simulink model "gm_fft_st"  (R2015a)
settings: Solver=ode45  StartTime=0.0  StopTime=1000.0  RelTol=1e-3
libraries: simulink x3, dspxfrm3 x1, hdlsllib x1
settings Model: CovSFcnEnable=off  Creator=tjia  LastModifiedBy=tjia
settings ConfigSet: ConfigType=Model
settings SolverCC: Priority=auto
settings OptimizationCC: BlockReduction=off  ConditionallyExecuteInputs=off  InlineParamsCompatibleMode=off  UseDivisionForNetSlopeComputation=Off  ForceBlockIOInitOptimize=off  EvaledLifeSpan=Inf  SimCompilerOptimization=Off
settings DebuggingCC: SolverPrmCheckMsg=warning  InheritedTsInSrcMsg=none  AllowSymbolicDim=off  SFMismatchInSimAndRtwBecauseOfMissingDataTypeDiag=warning
settings RTWCC: EnableTagging=off  RTWCompilerOptimization=Off
settings CodeAppCC: ParameterTuningSideEffectCode=Output function  AllmanStyle=off
settings GRTTargetCC: EnableShiftOperators=off  PortableWordSizesTransition=off  GenerateErtSFunctionTransition=off  CreateSILPILBlockTransition=None  CodeProfilingSaveOptionsTransition=SummaryOnly  CodeExecutionProfilingTransition=off  CodeProfilingInstrumentationTransition=off  CodeExecutionProfileVariableTransition=executionProfile  GenerateClassInterface=off

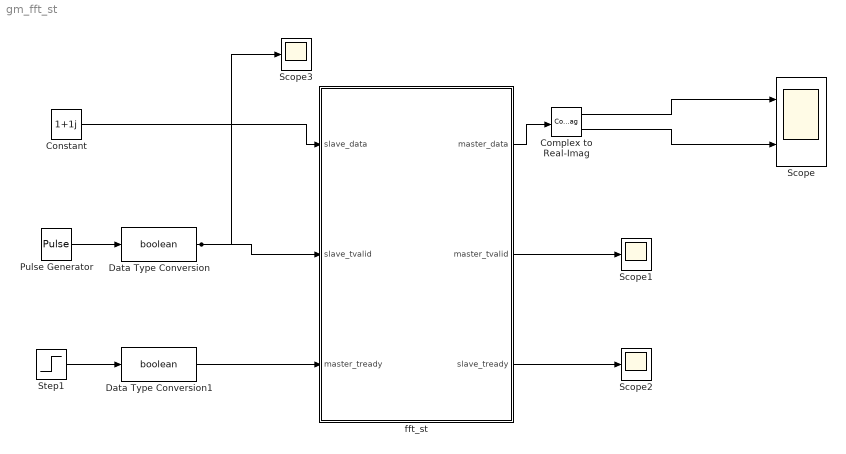
== system gm_fft_st ==
  Complex to Real-Imag : ComplexToRealImag  IOType=none  Commented=off  StatePerturbationForJacobian=1.0e-05
  Constant : Constant  IOType=none  Commented=off  StatePerturbationForJacobian=1.0e-05  Value=1+1j  OutDataTypeStr=int16  SampleTime=1
  Data Type Conversion : DataTypeConversion  IOType=none  Commented=off  StatePerturbationForJacobian=1.0e-05  OutDataTypeStr=boolean
  Data Type Conversion1 : DataTypeConversion  IOType=none  Commented=off  StatePerturbationForJacobian=1.0e-05  OutDataTypeStr=boolean
  Pulse Generator : DiscretePulseGenerator  IOType=none  Commented=off  StatePerturbationForJacobian=1.0e-05  Period=300  PulseWidth=64  PhaseDelay=236
  Scope : Scope  Commented=off  NumInputPorts=2
      settings: IOType=none  StatePerturbationForJacobian=1.0e-05  YMin=-5~-5  YMax=5~5
  Scope1 : Scope  Commented=off
      settings: IOType=none  StatePerturbationForJacobian=1.0e-05
  Scope2 : Scope  Commented=off
      settings: IOType=none  StatePerturbationForJacobian=1.0e-05  SaveName=ScopeData2
  Scope3 : Scope  Commented=off
      settings: IOType=none  StatePerturbationForJacobian=1.0e-05  SaveName=ScopeData3
  Step1 : Step  IOType=none  Commented=off  StatePerturbationForJacobian=1.0e-05  Time=200  SampleTime=1
  fft_st : Subsystem  IOType=none  Commented=off  StatePerturbationForJacobian=1.0e-05  TreatAsAtomicUnit=on
  wires:
  Step1/1 -> Data Type Conversion1/1
  fft_st/3(slave_tready) -> Scope2/1
  Data Type Conversion1/1 -> fft_st/3(master_tready)
  Complex to Real-Imag/2 -> Scope/2
  Complex to Real-Imag/1 -> Scope/1
  fft_st/1(master_data) -> Complex to Real-Imag/1
  Data Type Conversion/1 -> fft_st/2(slave_tvalid), Scope3/1
  fft_st/2(master_tvalid) -> Scope1/1
  Pulse Generator/1 -> Data Type Conversion/1
  Constant/1 -> fft_st/1(slave_data)

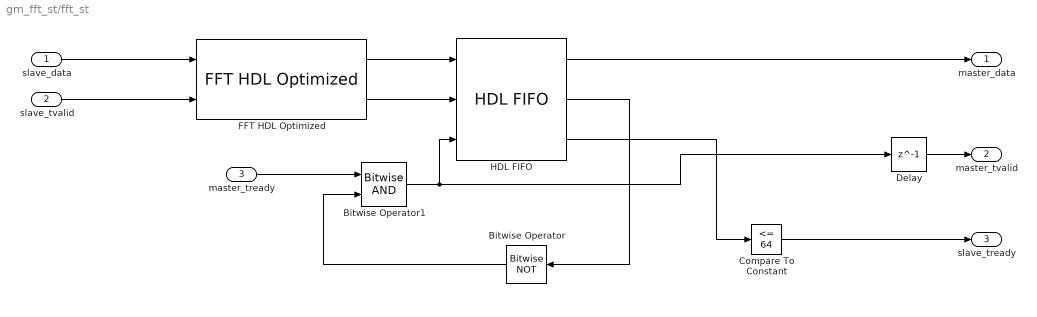
== system gm_fft_st/fft_st ==
  slave_data : Inport  IOType=none  Commented=off  StatePerturbationForJacobian=1.0e-05
  slave_tvalid : Inport  IOType=none  Commented=off  StatePerturbationForJacobian=1.0e-05  Port=2
  master_tready : Inport  IOType=none  Commented=off  StatePerturbationForJacobian=1.0e-05  Port=3
  Bitwise Operator : simulink/Logic and Bit Operations/Bitwise Operator  IOType=none  Commented=off  StatePerturbationForJacobian=1.0e-05  logicop=NOT  UseBitMask=off  BitMask=bin2dec('11011001')  BitMaskRealWorld=Stored Integer
  Bitwise Operator1 : simulink/Logic and Bit Operations/Bitwise Operator  IOType=none  Commented=off  StatePerturbationForJacobian=1.0e-05  logicop=AND  UseBitMask=off  NumInputPorts=2  BitMask=bin2dec('11011001')  BitMaskRealWorld=Stored Integer
  Compare To Constant : simulink/Logic and Bit Operations/Compare To Constant  IOType=none  Commented=off  StatePerturbationForJacobian=1.0e-05  relop=<=  const=64  OutDataTypeStr=boolean
  Delay : Delay  IOType=none  Commented=off  StatePerturbationForJacobian=1.0e-05  DelayLength=1  InitialCondition=0
  FFT HDL Optimized : dspxfrm3/FFT HDL Optimized  IOType=none  Commented=off  StatePerturbationForJacobian=1.0e-05  BitReversedOutput=off  Normalize=on  FFTLengthSource=Property  FFTLength=64  RoundingMethod=Floor  OverflowAction=Wrap  ValidInputPort=on  ResetInputPort=off  StartOutputPort=off  EndOutputPort=off  SimulateUsing=Code generation
  HDL FIFO : hdlsllib/HDL Operations/HDL FIFO  IOType=none  Commented=off  StatePerturbationForJacobian=1.0e-05  fifo_size=128  ratio=1  push_msg=Warning  pop_msg=Warning  show_empty=on  show_full=off  show_num=on
  master_data : Outport  IOType=none  Commented=off  StatePerturbationForJacobian=1.0e-05
  master_tvalid : Outport  IOType=none  Commented=off  StatePerturbationForJacobian=1.0e-05  Port=2
  slave_tready : Outport  IOType=none  Commented=off  StatePerturbationForJacobian=1.0e-05  Port=3
  wires:
  HDL FIFO/3 -> Compare To Constant/1
  Delay/1 -> master_tvalid/1
  Compare To Constant/1 -> slave_tready/1
  Bitwise Operator1/1 -> HDL FIFO/3, Delay/1
  Bitwise Operator/1 -> Bitwise Operator1/2
  master_tready/1 -> Bitwise Operator1/1
  HDL FIFO/2 -> Bitwise Operator/1
  FFT HDL Optimized/2 -> HDL FIFO/2
  HDL FIFO/1 -> master_data/1
  slave_data/1 -> FFT HDL Optimized/1
  slave_tvalid/1 -> FFT HDL Optimized/2
  FFT HDL Optimized/1 -> HDL FIFO/1
